simulink model "workshop7_simulink"  (R2023a)
settings: Solver=VariableStepAuto  StartTime=0.0  StopTime=10.0  RelTol=1e-3
settings Model: Creator=seanmcgowan  LastModifiedBy=seanmcgowan

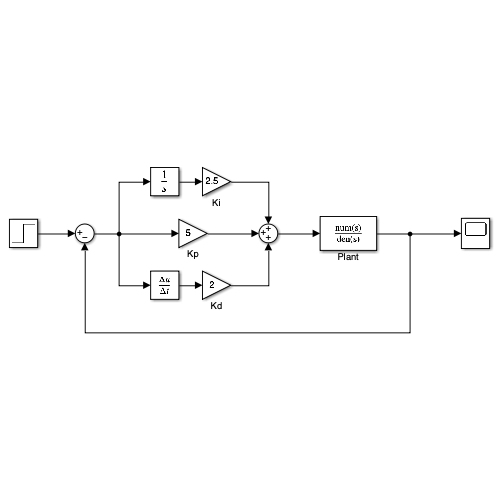
[thumbnail: Simulink's stored preview of the top-level diagram]
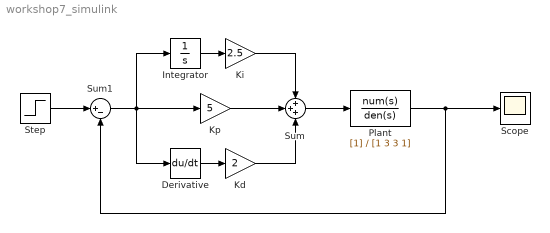
== system workshop7_simulink ==
  Derivative : Derivative
  Integrator : Integrator
  Kd : Gain  Gain=2
  Ki : Gain  Gain=2.5
  Kp : Gain  Gain=5
  Plant : TransferFcn  Denominator=[1 3 3 1]
  Scope : Scope
  Step : Step  Time=0  SampleTime=0
  Sum : Sum  Inputs=+++
  Sum1 : Sum  Inputs=|+-
  wires:
  Sum1/1 -> Derivative/1, Kp/1, Integrator/1
  Derivative/1 -> Kd/1
  Integrator/1 -> Ki/1
  Step/1 -> Sum1/1
  Plant/1 -> Sum1/2, Scope/1
  Kd/1 -> Sum/3
  Kp/1 -> Sum/2
  Ki/1 -> Sum/1
  Sum/1 -> Plant/1
